simulink model "master"  (R2020a)
settings: Solver=VariableStepAuto  StartTime=0.0  StopTime=40  RelTol=1e-9
values from neighbouring files (symbols this model uses):
  Theta_0 = 5    [variablen_ersteller.m]
settings Model: Creator=Alexander Grebien  LastModifiedBy=Alexander Grebien

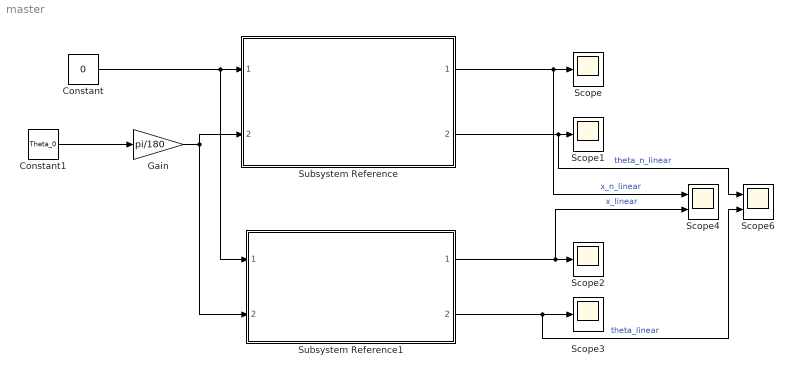
== system master ==
  Constant : Constant  Value=0
  Constant1 : Constant  Value=Theta_0
  Gain : Gain  Gain=pi/180
  Scope{,1..3} (4 alike) : Scope
  Scope4 : Scope  NumInputPorts=2
  Scope6 : Scope  NumInputPorts=2
  Subsystem Reference : Subsystem  ReferencedSubsystem=non_linear_model
  Subsystem Reference1 : Subsystem  ReferencedSubsystem=linearized_model
  wires:
  Constant1/1 -> Gain/1
  Constant/1 -> Subsystem Reference1/1, Subsystem Reference/1
  Subsystem Reference/2 -> Scope6/1, Scope1/1  "theta_n_linear"
  Subsystem Reference/1 -> Scope4/1, Scope/1  "x_n_linear"
  Gain/1 -> Subsystem Reference1/2, Subsystem Reference/2
  Subsystem Reference1/2 -> Scope6/2, Scope3/1  "theta_linear"
  Subsystem Reference1/1 -> Scope4/2, Scope2/1  "x_linear"
